simulink model "Multi_agent_system"  (R2016b)
settings: Solver=VariableStepAuto  StartTime=0.0  StopTime=100  RelTol=1e-3
values from neighbouring files (symbols this model uses):
  A = [ 0  0  3 ... (first row only)    [config.m]
  a = 1    [config.m]
  aa = 1    [config.m]
  b = [1 ... (first row only)    [config.m]
  bb = 1    [config.m]
  K = 1    [config.m]
  n = 3    [config.m]
  p = 0.5    [config.m]
  q = 1.5    [config.m]
  v = 0.5    [config.m]
  x_initial = x_initial*gain    [config.m]
  x_leader = x_leader*gain    (= 300)    [config.m]
settings Model: Creator=kvlton  LastModifiedBy=kvlton

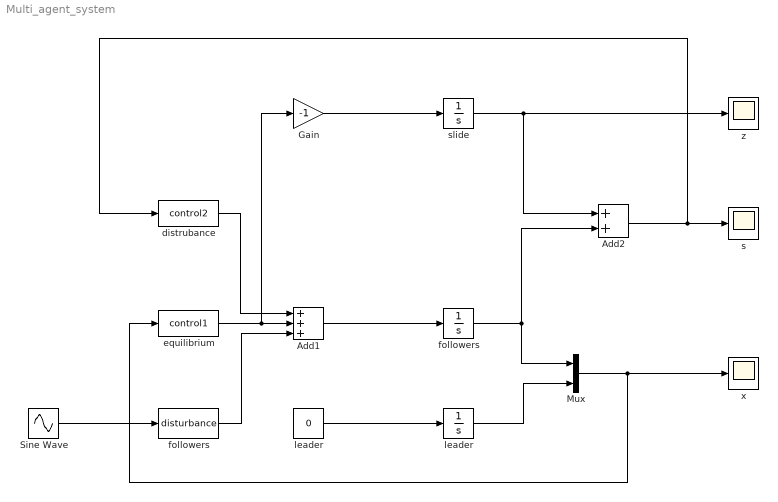
== system Multi_agent_system ==
  Add1 : Sum  Inputs=+++
  Add2 : Sum
  Gain : Gain  Gain=-1
  Mux : Mux  Inputs=2
  Sine Wave : Sin  SampleTime=0
  distrubance : S-Function  FunctionName=control2  Parameters=n,aa,bb,K,p,q  SFunctionDeploymentMode=off  EnableBusSupport=off
  equilibrium : S-Function  FunctionName=control1  Parameters=A,b,n,a,u,v  SFunctionDeploymentMode=off  EnableBusSupport=off
  followers : Integrator  InitialCondition=x_initial
  "followers " : S-Function  FunctionName=disturbance  Parameters=n  SFunctionDeploymentMode=off  EnableBusSupport=off
  leader : Integrator  InitialCondition=x_leader
  "leader " : Constant  Value=0
  s : Scope
  slide : Integrator  InitialCondition=x_initial*10
  x : Scope
  z : Scope
  wires:
  followers/1 -> Mux/1, Add2/2
  slide/1 -> z/1, Add2/1
  Add2/1 -> distrubance/1, s/1
  equilibrium/1 -> Add1/2, Gain/1
  "followers "/1 -> Add1/3
  Gain/1 -> slide/1
  distrubance/1 -> Add1/1
  "leader "/1 -> leader/1
  Add1/1 -> followers/1
  leader/1 -> Mux/2
  Mux/1 -> equilibrium/1, x/1
  Sine Wave/1 -> "followers "/1
